simulink model "Simple_Kalman_Filter"  (R2020a)
settings: Solver=FixedStepAuto  StartTime=0.0  StopTime=10.0  FixedStep=DT  RelTol=1e-3
values from neighbouring files (symbols this model uses):
  A_aug = [-C_d/J_r -K_d/(m*J_r) C_d/J_r s/J_r; m 0 -m 0; C_d/(g*J_g) K_d/(m*g*J_g) -C_d/(g*J_g) 0; 0 0 0 0]    [run_Top_Model.m]
  B_aug = [0; 0; -s/(g*J_g); 0]    [run_Top_Model.m]
  ini_torque = 0    [run_Top_Model.m]
  m = size(B, 2)    [eor_solve.m]    (also in regression.m = 2000; run_Top_Model.m = 1000)
  Omega_g_0 = 1    [run_Top_Model.m]
  Omega_r_0 = 1    [run_Top_Model.m]
  phi_0 = 0    [run_Top_Model.m]
  s = tf('s')    [baseline_design.m]    (also in eor_solve.m = size(S, 1); run_Top_Model.m = 1000000)
  tp = turbine_params_5MW()    [baseline_design.m]    (also in run_Top_Model.m)
undefined symbols (not defined in the file or in its folder): A_pitch, B_pitch, C_pitch, ini_pitch, L_kal_pitch, L_kalman
libraries: simulink x1
settings Model: Creator=lpwoolcock  LastModifiedBy=Vince

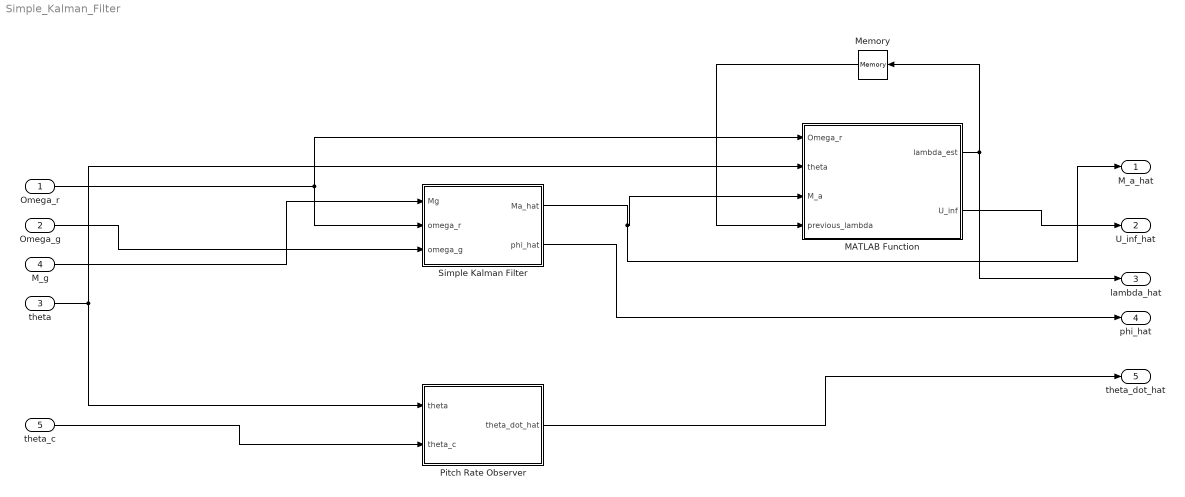
== system Simple_Kalman_Filter ==
  Omega_r : Inport
  Omega_g : Inport  Port=2
  theta : Inport  Port=3
  M_g : Inport  Port=4
  theta_c : Inport  Port=5
  MATLAB Function : MATLAB Function  TreatAsAtomicUnit=on
  Memory : Memory  InitialCondition=tp.lambda_star
  Pitch Rate Observer : Subsystem  TreatAsAtomicUnit=on
  Simple Kalman Filter : Subsystem  TreatAsAtomicUnit=on
  M_a_hat : Outport
  U_inf_hat : Outport  Port=2
  lambda_hat : Outport  Port=3
  phi_hat : Outport  Port=4
  theta_dot_hat : Outport  Port=5
  wires:
  M_g/1 -> Simple Kalman Filter/1(Mg)
  Omega_r/1 -> Simple Kalman Filter/2(omega_r), MATLAB Function/1(Omega_r)
  Omega_g/1 -> Simple Kalman Filter/3(omega_g)
  Memory/1 -> MATLAB Function/4(previous_lambda)
  MATLAB Function/1(lambda_est) -> lambda_hat/1, Memory/1
  Simple Kalman Filter/1(Ma_hat) -> M_a_hat/1, MATLAB Function/3(M_a)
  theta/1 -> Pitch Rate Observer/1(theta), MATLAB Function/2(theta)
  MATLAB Function/2(U_inf) -> U_inf_hat/1
  theta_c/1 -> Pitch Rate Observer/2(theta_c)
  Simple Kalman Filter/2(phi_hat) -> phi_hat/1
  Pitch Rate Observer/1(theta_dot_hat) -> theta_dot_hat/1

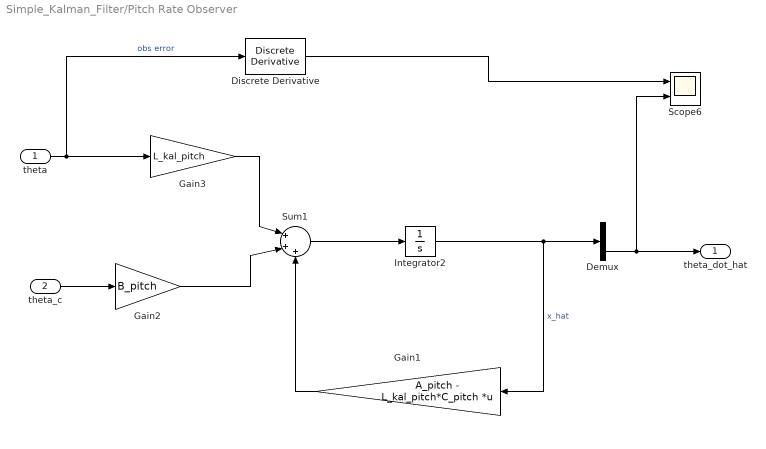
== system Simple_Kalman_Filter/Pitch Rate Observer ==
  theta : Inport
  theta_c : Inport  Port=2
  Demux : Demux  Outputs=2
  Discrete Derivative : simulink/Discrete/Discrete Derivative  gainval=1.0  ICPrevScaledInput=0.0  OutMin=[]  OutMax=[]  OutDataType=fixdt(1, 16)  OutScaling=2^-10  DoSatur=off
  Gain1 : Gain  Gain=A_pitch - L_kal_pitch*C_pitch  Multiplication=Matrix(K*u)
  Gain2 : Gain  Gain=B_pitch
  Gain3 : Gain  Gain=L_kal_pitch
  Integrator2 : Integrator  InitialCondition=ini_pitch
  Scope6 : Scope  NumInputPorts=2
  Sum1 : Sum  Inputs=|+++
  theta_dot_hat : Outport
  wires:
  Sum1/1 -> Integrator2/1
  Gain2/1 -> Sum1/2
  Gain3/1 -> Sum1/1
  Integrator2/1 -> Gain1/1, Demux/1  "x_hat"
  theta/1 -> Discrete Derivative/1, Gain3/1  "obs error"
  Gain1/1 -> Sum1/3
  theta_c/1 -> Gain2/1
  Demux/2 -> Scope6/2, theta_dot_hat/1
  Discrete Derivative/1 -> Scope6/1

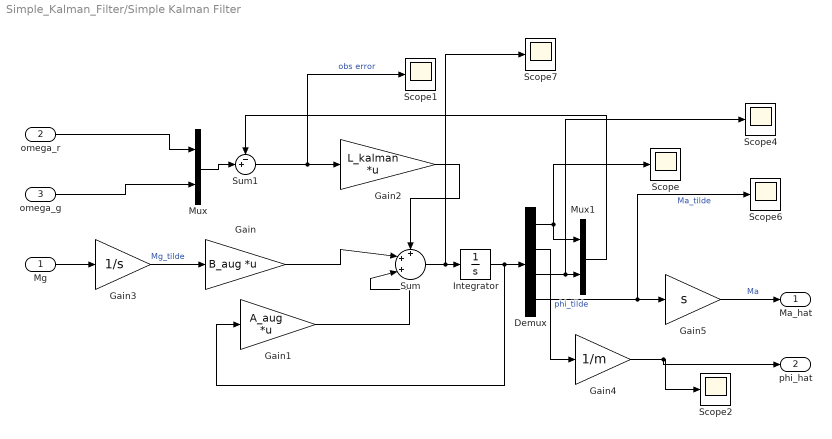
== system Simple_Kalman_Filter/Simple Kalman Filter ==
  Mg : Inport
  omega_r : Inport  Port=2
  omega_g : Inport  Port=3
  Demux : Demux
  Gain : Gain  Gain=B_aug  Multiplication=Matrix(K*u) (u vector)
  Gain1 : Gain  Gain=A_aug  Multiplication=Matrix(K*u) (u vector)
  Gain2 : Gain  Gain=L_kalman  Multiplication=Matrix(K*u) (u vector)
  Gain3 : Gain  Gain=1/s
  Gain4 : Gain  Gain=1/m
  Gain5 : Gain  Gain=s
  Integrator : Integrator  InitialCondition=[Omega_r_0; Omega_g_0; phi_0; ini_torque]
  Mux : Mux  Inputs=2
  Mux1 : Mux  Inputs=2
  Scope{,1..2,4,6..7} (6 alike) : Scope
  Sum : Sum  Inputs=+++|
  Sum1 : Sum  Inputs=-+|
  Ma_hat : Outport
  phi_hat : Outport  Port=2
  wires:
  Mg/1 -> Gain3/1
  omega_r/1 -> Mux/1
  omega_g/1 -> Mux/2
  Mux/1 -> Sum1/2
  Sum1/1 -> Scope1/1, Gain2/1  "obs error"
  Integrator/1 -> Gain1/1, Demux/1
  Demux/4 -> Scope6/1, Gain5/1  "Ma_tilde"
  Gain/1 -> Sum/2
  Gain1/1 -> Sum/3
  Sum/1 -> Scope7/1, Integrator/1
  Demux/3 -> Scope4/1, Mux1/2
  Demux/1 -> Scope/1, Mux1/1
  Mux1/1 -> Sum1/1
  Demux/2 -> Gain4/1  "phi_tilde"
  Gain3/1 -> Gain/1  "Mg_tilde"
  Gain5/1 -> Ma_hat/1  "Ma"
  Gain2/1 -> Sum/1
  Gain4/1 -> phi_hat/1, Scope2/1

== matlab function Simple_Kalman_Filter/MATLAB Function ==
  data: Omega_r input; theta input; lambda_est output; M_a input; U_inf output; tp parameter Bus: slBus1; previous_lambda input
% Computes the windspeed using a secant method with given torque
% estimation, rotor speed, and blade pitch angle
function [lambda_est, U_inf] = torque_to_windspeed(Omega_r, theta, M_a, tp, previous_lambda)

% constant in the equation Cp/lambda^3 = C
C = 2*M_a/(tp.rho*pi*(tp.R)^5*(Omega_r)^2);

% Now find the root of f(lambda) = Cp/lambda^3 - C
f = @(lambda) interp2(tp.theta_grid, tp.lambda_grid, tp.C_p, theta, lambda, 'cubic')/(lambda^3) - C;

% Initial guess is previous lambda value
[lambda_est, FVAL, EXITFLAG] = fzero(f, previous_lambda);

% couldn't find valid root, just use optimal lambda for Region 2
if EXITFLAG == -3
    lambda_est = tp.lambda_star; 
end

U_inf = tp.R*Omega_r/lambda_est;

end
